simulink model "Problem3"  (R2020b)
settings: Solver=VariableStepAuto  StartTime=0.0  StopTime=25  RelTol=1e-3
values from neighbouring files (symbols this model uses):
  ctrl = 1    [Init.m]
  g = 32.18    [Init.m]
  I = 5    [Init.m]
  Kf = 1    [Init.m]
  m = 50    [Init.m]
  mu = [0 .4 .8 .97 1.0 .98 .96 .94 .92 .9 .88 .855 .83 .81 .79 .77 .75 .73 .72 .71 .7]    [Init.m]
  PBmax = 1500    [Init.m]
  Rr = 15/12    (= 1.25)    [Init.m]
  slip = (0:.05:1.0)    [Init.m]
  TB = 0.01    [Init.m]
  v0 = 88    [Init.m]
settings Model: OrderedModelArguments=off  Creator=HP  LastModifiedBy=HP

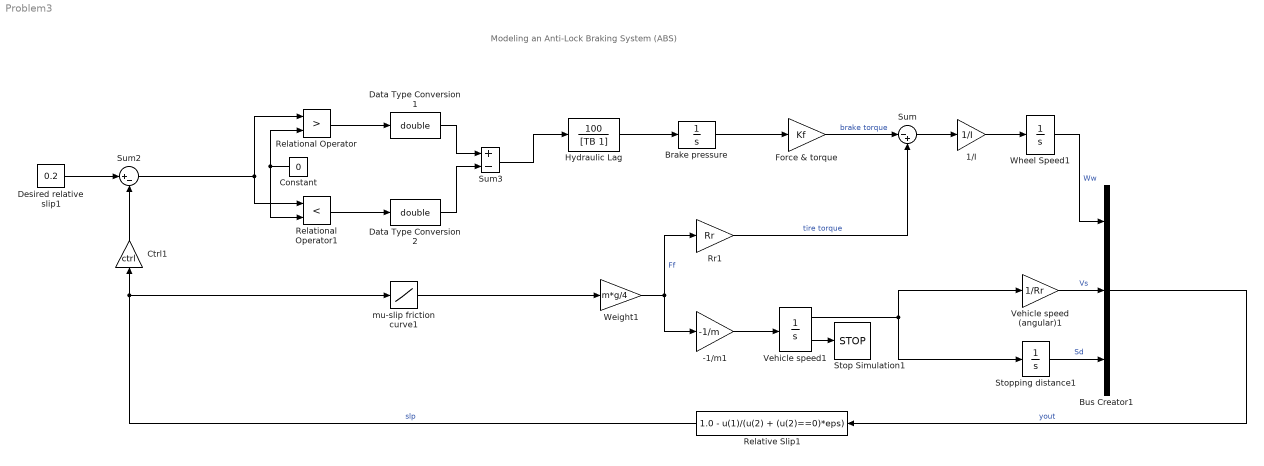
== system Problem3 ==
  note: Modeling an Anti-Lock Braking System (ABS)
  -1/m1 : Gain  Gain=-1/m  SaturateOnIntegerOverflow=on  OutDataTypeStr=Inherit: Same as input  ParamDataTypeStr=Inherit: Same as input
  1/I : Gain  Gain=1/I  SaturateOnIntegerOverflow=on  OutDataTypeStr=Inherit: Same as input  ParamDataTypeStr=Inherit: Same as input
  Brake pressure : Integrator  LimitOutput=on  UpperSaturationLimit=PBmax  LowerSaturationLimit=0
  Bus Creator1 : BusCreator  Inputs=3
  Constant : Constant  Value=0
  Ctrl1 : Gain  Gain=ctrl  SaturateOnIntegerOverflow=on  OutDataTypeStr=Inherit: Same as input  ParamDataTypeStr=Inherit: Same as input
  Data Type Conversion1 : DataTypeConversion  OutDataTypeStr=double  SaturateOnIntegerOverflow=on  RndMeth=Zero
  Data Type Conversion2 : DataTypeConversion  OutDataTypeStr=double  SaturateOnIntegerOverflow=on  RndMeth=Zero
  Desired relative slip1 : Constant  Value=0.2
  Force & torque : Gain  Gain=Kf  SaturateOnIntegerOverflow=on  OutDataTypeStr=Inherit: Same as input  ParamDataTypeStr=Inherit: Same as input
  "Hydraulic Lag " : TransferFcn  Numerator=[100]  Denominator=[TB 1]
  Relational Operator : RelationalOperator  Operator=>  OutDataTypeStr=boolean  RndMeth=Nearest  InputSameDT=on
  Relational Operator1 : RelationalOperator  Operator=<  OutDataTypeStr=boolean  RndMeth=Nearest  InputSameDT=on
  Relative Slip1 : Fcn  Expr=1.0 - u(1)/(u(2) + (u(2)==0)*eps)
  Rr1 : Gain  Gain=Rr  SaturateOnIntegerOverflow=on  OutDataTypeStr=Inherit: Same as input  ParamDataTypeStr=Inherit: Same as input
  Stop Simulation1 : Stop
  Stopping distance1 : Integrator  UpperSaturationLimit=1000  LowerSaturationLimit=0
  Sum : Sum  Inputs=|-+  InputSameDT=on  SaturateOnIntegerOverflow=on  OutDataTypeStr=Inherit: Same as first input
  Sum2 : Sum  Inputs=|+-  InputSameDT=on  SaturateOnIntegerOverflow=on  OutDataTypeStr=Inherit: Same as first input
  Sum3 : Sum  Inputs=+-  InputSameDT=on  SaturateOnIntegerOverflow=on  OutDataTypeStr=Inherit: Same as first input
  Vehicle speed1 : Integrator  InitialCondition=v0  LimitOutput=on  UpperSaturationLimit=1000  LowerSaturationLimit=0  ShowSaturationPort=on
  Vehicle speed (angular)1 : Gain  Gain=1/Rr  SaturateOnIntegerOverflow=on  OutDataTypeStr=Inherit: Same as input  ParamDataTypeStr=Inherit: Same as input
  Weight1 : Gain  Gain=m*g/4  SaturateOnIntegerOverflow=on  OutDataTypeStr=Inherit: Same as input  ParamDataTypeStr=Inherit: Same as input
  Wheel Speed1 : Integrator  InitialCondition=v0/Rr  LimitOutput=on  UpperSaturationLimit=1000  LowerSaturationLimit=0
  mu-slip friction curve1 : Lookup_n-D  NumberOfTableDimensions=1  BreakpointsForDimension1=slip  Table=mu  SaturateOnIntegerOverflow=on  InputSameDT=on
  wires:
  Desired relative slip1/1 -> Sum2/1
  Ctrl1/1 -> Sum2/2
  Sum/1 -> 1/I/1
  Wheel Speed1/1 -> Bus Creator1/1  "Ww"
  Sum3/1 -> "Hydraulic Lag "/1
  Force & torque/1 -> Sum/1  "brake torque"
  "Hydraulic Lag "/1 -> Brake pressure/1
  Brake pressure/1 -> Force & torque/1
  1/I/1 -> Wheel Speed1/1
  -1/m1/1 -> Vehicle speed1/1
  mu-slip friction curve1/1 -> Weight1/1
  Rr1/1 -> Sum/2  "tire torque"
  Weight1/1 -> -1/m1/1, Rr1/1  "Ff"
  Vehicle speed1/1 -> Stopping distance1/1, Vehicle speed (angular)1/1
  Vehicle speed1/2 -> Stop Simulation1/1
  Stopping distance1/1 -> Bus Creator1/3  "Sd"
  Vehicle speed (angular)1/1 -> Bus Creator1/2  "Vs"
  Bus Creator1/1 -> Relative Slip1/1  "yout"
  Relative Slip1/1 -> Ctrl1/1, mu-slip friction curve1/1  "slp"
  Data Type Conversion2/1 -> Sum3/2
  Relational Operator1/1 -> Data Type Conversion2/1
  Relational Operator/1 -> Data Type Conversion1/1
  Data Type Conversion1/1 -> Sum3/1
  Constant/1 -> Relational Operator1/2, Relational Operator/2
  Sum2/1 -> Relational Operator/1, Relational Operator1/1
